simulink model "commandABT"  (R2023a)
settings: Solver=FixedStepAuto  StartTime=0.0  StopTime=inf  RelTol=1e-3  EnableMultiTasking=on
undefined symbols (not defined in the file or in its folder): Aw, I, Kp, Kpd, PWMcmdMono1, PWMcmdMono2, PWMcmdMono3, PWMcmdMono4, speedMono1, speedMono2, speedMono3, speedMono4
libraries: arduinolib x8, arduinosensorlib x2, sharedtransform x2, mspfiltlib x1, matrix_library x1
settings Model: ExtModeTrigDuration=2  Creator=C23Clement.Azpiroz.F  LastModifiedBy=Clément
settings OptimizationCC: EnhancedBackFolding=on  PassReuseOutputArgsAs=Individual arguments  ZeroExternalMemoryAtStartup=off  ZeroInternalMemoryAtStartup=off  MaxStackSize=64  OptimizeBlockOrder=speed  DifferentSizesBufferReuse=on  OptimizationCustomize=off  EfficientTunableParamExpr=on
settings DebuggingCC: ParameterTunabilityLossMsg=error
settings HardwareCC: ProdBitPerPointer=32  ProdBitPerSizeT=32  ProdBitPerPtrDiffT=32  ProdLargestAtomicInteger=Long  ProdLargestAtomicFloat=Double  ProdWordSize=32  ProdHWDeviceType=ARM Compatible->ARM Cortex  UseEmbeddedCoderFeatures=off
settings SFSimCC: MATLABDynamicMemAlloc=off
settings RTWCC: Description=Embedded Coder  SystemTargetFile=ert.tlc  HardwareBoard=Arduino MKR1000  TemplateMakefile=ert_default_tmf  Toolchain=Arduino ARM  BuildConfiguration=Faster Runs
settings CodeAppCC: ForceParamTrailComments=on  OperatorAnnotations=on  SimulinkDataObjDesc=on  SFDataObjDesc=on  InsertBlockDesc=on
settings ERTTargetCC: SupportContinuousTime=on  SupportNonInlinedSFcns=on  SupportVariableSizeSignals=on  ExtModeTransport=2  ExtModeStaticAlloc=on  ExtModeAutomaticAllocSize=off  ExtModeStaticAllocSize=8192  ExtModeMexFile=ext_xcp  ExtModeIntrfLevel=Level2 - Open  ERTSrcFileBannerTemplate=codertarget_code_template.cgt  ERTHdrFileBannerTemplate=codertarget_code_template.cgt  ERTDataSrcFileTemplate=codertarget_code_template.cgt  ERTDataHdrFileTemplate=codertarget_code_template.cgt

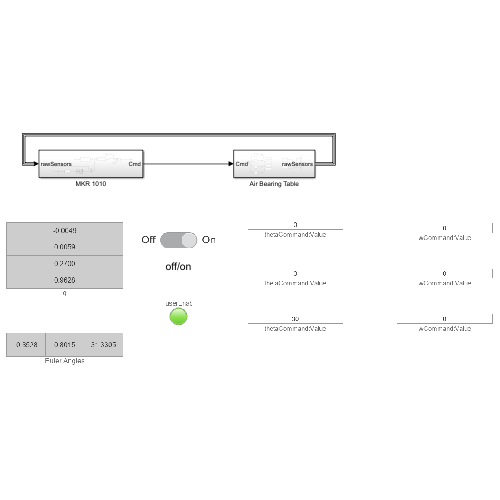
[thumbnail: Simulink's stored preview of the top-level diagram]
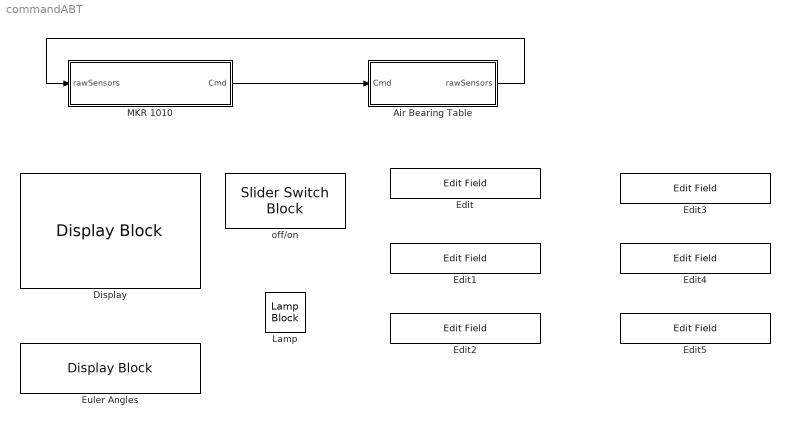
== system commandABT ==
  Air Bearing Table : Subsystem
  Display : DisplayBlock  LabelPosition=Bottom  Transparency=1
  Edit{,1..5} (6 alike) : EditField  LabelPosition=Bottom  ShowInitialText=on  Alignment=Center
  Euler Angles : DisplayBlock  LabelPosition=Bottom  Transparency=1
  Lamp : LampBlock
  MKR 1010 : Subsystem
  off/on : SliderSwitchBlock  LabelPosition=Hide
      settings: Values={{'Off', 'On'}, [0 1]}
  wires:
  Air Bearing Table/1(rawSensors) -> MKR 1010/1(rawSensors)
  MKR 1010/1(Cmd) -> Air Bearing Table/1(Cmd)

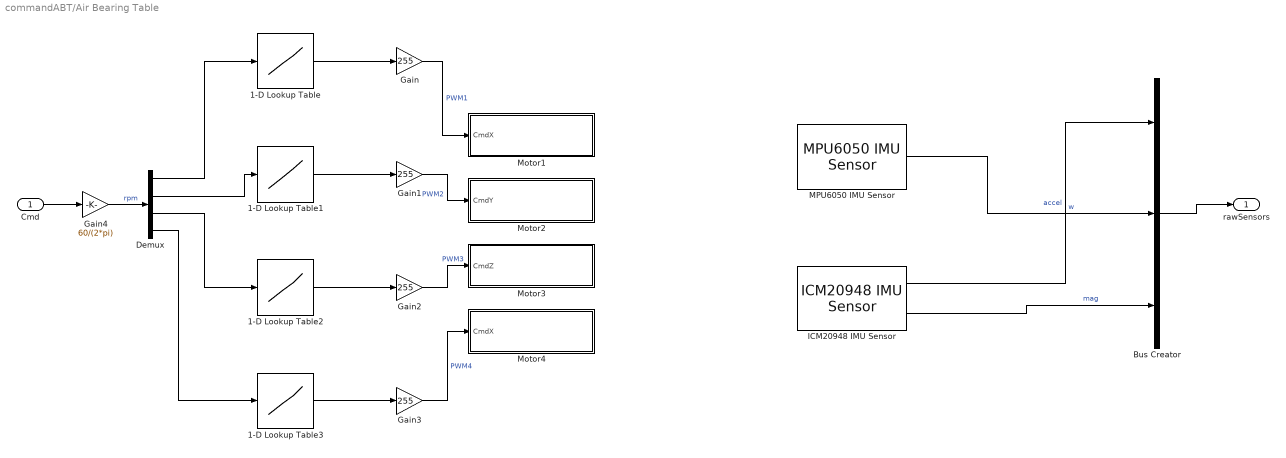
== system commandABT/Air Bearing Table ==
  Cmd : Inport
  1-D Lookup Table : Lookup_n-D  NumberOfTableDimensions=1  BreakpointsForDimension1=speedMono1  Table=PWMcmdMono1  InternalRulePriority=Speed  RndMeth=Simplest
  1-D Lookup Table1 : Lookup_n-D  NumberOfTableDimensions=1  BreakpointsForDimension1=speedMono2  Table=PWMcmdMono2  InternalRulePriority=Speed  RndMeth=Simplest
  1-D Lookup Table2 : Lookup_n-D  NumberOfTableDimensions=1  BreakpointsForDimension1=speedMono3  Table=PWMcmdMono3  InternalRulePriority=Speed  RndMeth=Simplest
  1-D Lookup Table3 : Lookup_n-D  NumberOfTableDimensions=1  BreakpointsForDimension1=speedMono4  Table=PWMcmdMono4  InternalRulePriority=Speed  RndMeth=Simplest
  Bus Creator : BusCreator  Inputs=3
  Demux : Demux
  Gain{,1..3} (4 alike) : Gain  Gain=255
  Gain4 : Gain  Gain=60/(2*pi)
  ICM20948 IMU Sensor : arduinosensorlib/ICM20948 IMU Sensor  I2CAddress=0x69  BitRate=1000000  EnableDRDY=off  InterruptType=Active high  IsActiveAccel=on  IsActiveGyro=off  IsActiveMag=on  IsActiveTemp=off  IsActiveStatus=off  IsActiveTimeStamp=off  AccelerometerRange=+/-2g  AccelerometerODR=1125  AccelerometerBW=23.9 Hz  GyroscopeRange=+/-250 dps  GyroscopeODR=1125  GyroscopeBW=23.9 Hz  MagnetometerODR=100 Hz  TemperatureBW=34.1 Hz  DataType=double  spf=1  SampleTime=0.1  QueueSizeFactor=1
  MPU6050 IMU Sensor : arduinosensorlib/MPU6050 IMU Sensor  SlaveAddress=0x68  Accel=off  AngularRate=on  Temperature=off  Status=off  Timestamp=off  EulerAngles=off  Quat=off  AccelRange=2G  GyroRange=250 dps  DmpOdr=200 Hz  Dlpf=Accelerometer: 184Hz, Gyroscope: 188Hz  spf=1  SampleTime=0.1  QueueSizeFactor=1
  Motor1 : Subsystem
  Motor2 : Subsystem
  Motor3 : Subsystem
  Motor4 : Subsystem
  rawSensors : Outport
  wires:
  Bus Creator/1 -> rawSensors/1
  Demux/1 -> 1-D Lookup Table/1
  Gain/1 -> Motor1/1(CmdX)  "PWM1"
  Cmd/1 -> Gain4/1
  1-D Lookup Table2/1 -> Gain2/1
  1-D Lookup Table1/1 -> Gain1/1
  Gain4/1 -> Demux/1  "rpm"
  Gain2/1 -> Motor3/1(CmdZ)  "PWM3"
  Gain3/1 -> Motor4/1(CmdX)  "PWM4"
  Demux/4 -> 1-D Lookup Table3/1
  Demux/3 -> 1-D Lookup Table2/1
  1-D Lookup Table/1 -> Gain/1
  Gain1/1 -> Motor2/1(CmdY)  "PWM2"
  Demux/2 -> 1-D Lookup Table1/1
  1-D Lookup Table3/1 -> Gain3/1
  MPU6050 IMU Sensor/1 -> Bus Creator/2  "w"
  ICM20948 IMU Sensor/1 -> Bus Creator/1  "accel"
  ICM20948 IMU Sensor/2 -> Bus Creator/3  "mag"

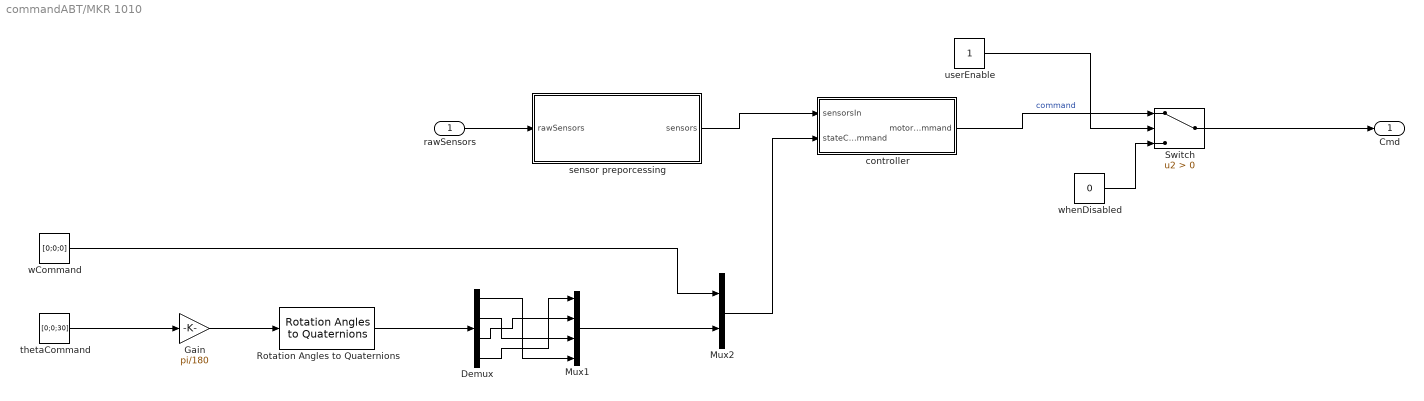
== system commandABT/MKR 1010 ==
  rawSensors : Inport
  Demux : Demux
  Gain : Gain  Gain=pi/180
  Mux1 : Mux
  Mux2 : Mux  Inputs=2
  Rotation Angles to Quaternions : sharedtransform/Rotation Angles to Quaternions  rotationOrder=ZYX  aMode=aMode
  Switch : Switch  Criteria=u2 > Threshold  SaturateOnIntegerOverflow=off  InputSameDT=off
  controller : Subsystem
  sensor preporcessing : Subsystem
  thetaCommand : Constant  Value=[0;0;30]
  userEnable : Constant
  wCommand : Constant  Value=[0;0;0]
  whenDisabled : Constant  Value=0
  Cmd : Outport
  wires:
  rawSensors/1 -> sensor preporcessing/1(rawSensors)
  userEnable/1 -> Switch/2
  sensor preporcessing/1(sensors) -> controller/1(sensorsIn)
  whenDisabled/1 -> Switch/3
  controller/1(motorCommand) -> Switch/1  "command"
  Switch/1 -> Cmd/1
  Demux/1 -> Mux1/4
  Demux/4 -> Mux1/1
  Demux/2 -> Mux1/3
  Demux/3 -> Mux1/2
  Gain/1 -> Rotation Angles to Quaternions/1
  Rotation Angles to Quaternions/1 -> Demux/1
  thetaCommand/1 -> Gain/1
  wCommand/1 -> Mux2/1
  Mux1/1 -> Mux2/2
  Mux2/1 -> controller/2(stateCommand)

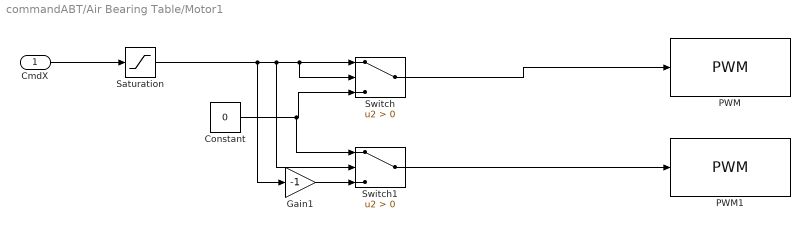
== system commandABT/Air Bearing Table/Motor1 ==
  CmdX : Inport
  Constant : Constant  Value=0
  Gain1 : Gain  Gain=-1
  PWM : arduinolib/PWM  pinNumber=2  frequencyType=Default  desiredFrequency=490.2  achievableFrequency=490.2
  PWM1 : arduinolib/PWM  pinNumber=3  frequencyType=Default  desiredFrequency=490.2  achievableFrequency=490.2
  Saturation : Saturate  UpperLimit=255  LowerLimit=-255
  Switch : Switch  Criteria=u2 > Threshold  SaturateOnIntegerOverflow=off  InputSameDT=off
  Switch1 : Switch  Criteria=u2 > Threshold  SaturateOnIntegerOverflow=off  InputSameDT=off
  wires:
  Switch1/1 -> PWM1/1
  CmdX/1 -> Saturation/1
  Switch/1 -> PWM/1
  Saturation/1 -> Gain1/1, Switch/1, Switch/2, Switch1/2
  Constant/1 -> Switch1/1, Switch/3
  Gain1/1 -> Switch1/3

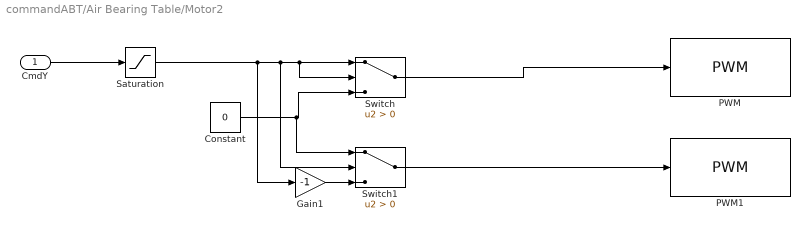
== system commandABT/Air Bearing Table/Motor2 ==
  CmdY : Inport
  Constant : Constant  Value=0
  Gain1 : Gain  Gain=-1
  PWM : arduinolib/PWM  pinNumber=4  frequencyType=Default  desiredFrequency=490.2  achievableFrequency=490.2
  PWM1 : arduinolib/PWM  pinNumber=5  frequencyType=Default  desiredFrequency=490.2  achievableFrequency=490.2
  Saturation : Saturate  UpperLimit=255  LowerLimit=-255
  Switch : Switch  Criteria=u2 > Threshold  SaturateOnIntegerOverflow=off  InputSameDT=off
  Switch1 : Switch  Criteria=u2 > Threshold  SaturateOnIntegerOverflow=off  InputSameDT=off
  wires:
  Switch1/1 -> PWM1/1
  CmdY/1 -> Saturation/1
  Switch/1 -> PWM/1
  Saturation/1 -> Gain1/1, Switch/1, Switch/2, Switch1/2
  Constant/1 -> Switch1/1, Switch/3
  Gain1/1 -> Switch1/3

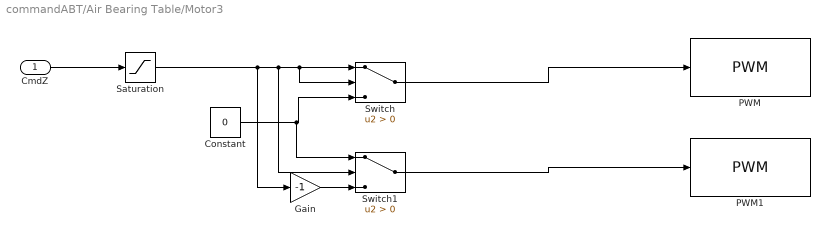
== system commandABT/Air Bearing Table/Motor3 ==
  CmdZ : Inport
  Constant : Constant  Value=0
  Gain : Gain  Gain=-1
  PWM : arduinolib/PWM  pinNumber=0  frequencyType=Default  desiredFrequency=490.2  achievableFrequency=490.2
  PWM1 : arduinolib/PWM  pinNumber=1  frequencyType=Default  desiredFrequency=490.2  achievableFrequency=490.2
  Saturation : Saturate  UpperLimit=255  LowerLimit=-255
  Switch : Switch  Criteria=u2 > Threshold  SaturateOnIntegerOverflow=off  InputSameDT=off
  Switch1 : Switch  Criteria=u2 > Threshold  SaturateOnIntegerOverflow=off  InputSameDT=off
  wires:
  Switch1/1 -> PWM1/1
  CmdZ/1 -> Saturation/1
  Switch/1 -> PWM/1
  Constant/1 -> Switch1/1, Switch/3
  Saturation/1 -> Gain/1, Switch1/2, Switch/2, Switch/1
  Gain/1 -> Switch1/3

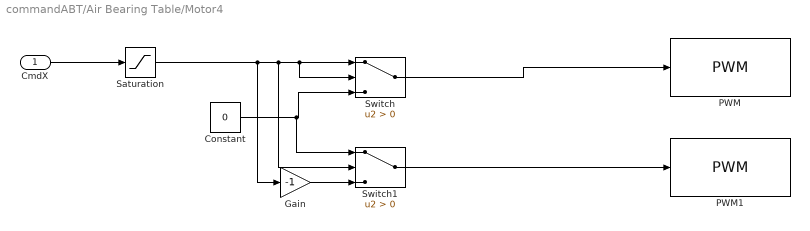
== system commandABT/Air Bearing Table/Motor4 ==
  CmdX : Inport
  Constant : Constant  Value=0
  Gain : Gain  Gain=-1
  PWM : arduinolib/PWM  pinNumber=6  frequencyType=Default  desiredFrequency=490.2  achievableFrequency=490.2
  PWM1 : arduinolib/PWM  pinNumber=7  frequencyType=Default  desiredFrequency=490.2  achievableFrequency=490.2
  Saturation : Saturate  UpperLimit=255  LowerLimit=-255
  Switch : Switch  Criteria=u2 > Threshold  SaturateOnIntegerOverflow=off  InputSameDT=off
  Switch1 : Switch  Criteria=u2 > Threshold  SaturateOnIntegerOverflow=off  InputSameDT=off
  wires:
  Switch1/1 -> PWM1/1
  CmdX/1 -> Saturation/1
  Switch/1 -> PWM/1
  Constant/1 -> Switch1/1, Switch/3
  Saturation/1 -> Gain/1, Switch1/2, Switch/2, Switch/1
  Gain/1 -> Switch1/3

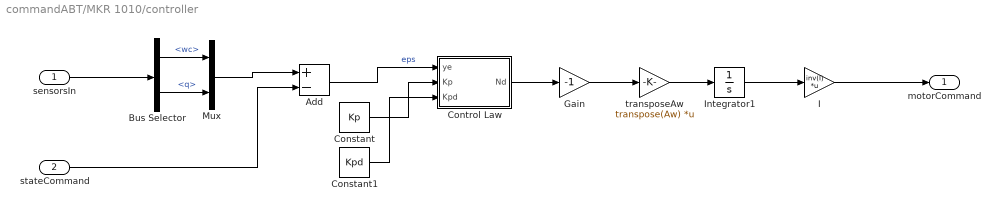
== system commandABT/MKR 1010/controller ==
  sensorsIn : Inport
  stateCommand : Inport  Port=2
  Add : Sum  Inputs=+-
  Bus Selector : BusSelector  OutputSignals=wc,q
  Constant : Constant  Value=Kp
  Constant1 : Constant  Value=Kpd
  Control Law : MATLAB Function  TreatAsAtomicUnit=on
  Gain : Gain  Gain=-1
  I : Gain  Gain=inv(I)  Multiplication=Matrix(K*u)
  Integrator1 : Integrator  InitialCondition=[0.01; 0.01; 0.01; 0.01]
  Mux : Mux  Inputs=2
  transposeAw : Gain  Gain=transpose(Aw)  Multiplication=Matrix(K*u)
  motorCommand : Outport
  wires:
  sensorsIn/1 -> Bus Selector/1
  Bus Selector/1 -> Mux/1  "<wc>"
  Bus Selector/2 -> Mux/2  "<q>"
  Mux/1 -> Add/1
  stateCommand/1 -> Add/2
  Add/1 -> Control Law/1(ye)  "eps"
  Constant/1 -> Control Law/2(Kp)
  Constant1/1 -> Control Law/3(Kpd)
  Control Law/1(Nd) -> Gain/1
  transposeAw/1 -> Integrator1/1
  Integrator1/1 -> I/1
  I/1 -> motorCommand/1
  Gain/1 -> transposeAw/1

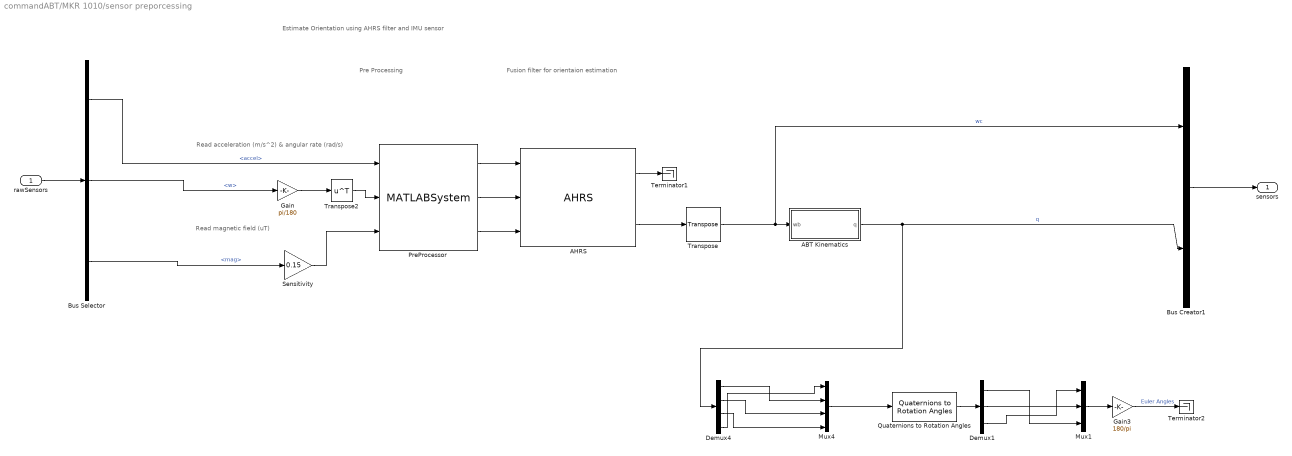
== system commandABT/MKR 1010/sensor preporcessing ==
  note: Fusion filter for orientaion estimation
  note: Read  acceleration (m/s^2) &
      | angular rate (rad/s)
  note: Read magnetic field (uT)
  note: Estimate Orientation using AHRS filter and IMU sensor
  note: Pre Processing
  rawSensors : Inport
  ABT Kinematics : Subsystem
  AHRS : mspfiltlib/AHRS  DispRefFrame=ENU  DecimationFactor=1  InitialProcessNoise=ahrsfilter.defaultProcessNoise  OrientationFormat=quaternion  SimulateUsing=Interpreted execution  AccelerometerNoise=0.000134  GyroscopeNoise=1.38347e-6  MagnetometerNoise=0.45  GyroscopeDriftNoise=0.1e-30  LinearAccelerationNoise=0.0096236100000000012  MagneticDisturbanceNoise=0.5  LinearAccelerationDecayFactor=0.5  MagneticDisturbanceDecayFactor=0.5  ExpectedMagneticFieldStrength=50
  Bus Creator1 : BusCreator  Inputs=2
  Bus Selector : BusSelector  OutputSignals=accel,w,mag
  Demux1 : Demux  Outputs=3
  Demux4 : Demux
  Gain : Gain  Gain=pi/180
  Gain3 : Gain  Gain=180/pi
  Mux1 : Mux  Inputs=3
  Mux4 : Mux
  PreProcessor : MATLABSystem  System=PreProcessor  MagOffsets=[-3.7477,2.6230,9.3852]  AccelXAxisIndex=2  AccelXAxisSign=-  AccelYAxisIndex=1  AccelYAxisSign=-  AccelZAxisIndex=3  AccelZAxisSign=-  GyroXAxisIndex=2  GyroXAxisSign=+  GyroYAxisIndex=1  GyroYAxisSign=-  GyroZAxisIndex=3  GyroZAxisSign=+  MagXAxisIndex=2  MagXAxisSign=-  MagYAxisIndex=1  MagYAxisSign=-  MagZAxisIndex=3  MagZAxisSign=-
      mask Type: PreProcessor
      mask Display:
      | disp('PreProcessor');
      | port_label('input',1,'accel');
      | port_label('input',2,'gyro');
      | port_label('input',3,'mag');
      | port_label('output',1,'accel');
      | port_label('output',2,'gyro');
      | port_label('output',3,'mag');
  Quaternions to Rotation Angles : sharedtransform/Quaternions to Rotation Angles  rotationOrder=ZYX  aMode=aMode
  Sensitivity : Gain  Gain=0.15  OutDataTypeStr=double  LockScale=on
  Terminator1 : Terminator
  Terminator2 : Terminator
  Transpose : matrix_library/Transpose
  Transpose2 : Math  Operator=transpose
  sensors : Outport
  wires:
  rawSensors/1 -> Bus Selector/1
  Bus Creator1/1 -> sensors/1
  Demux1/1 -> Mux1/3
  Demux1/3 -> Mux1/1
  Mux1/1 -> Gain3/1
  Quaternions to Rotation Angles/1 -> Demux1/1
  ABT Kinematics/1(q) -> Bus Creator1/2, Demux4/1  "q"
  Demux1/2 -> Mux1/2
  Gain3/1 -> Terminator2/1  "Euler Angles"
  Demux4/1 -> Mux4/2
  Demux4/3 -> Mux4/4
  Demux4/4 -> Mux4/1
  Demux4/2 -> Mux4/3
  Mux4/1 -> Quaternions to Rotation Angles/1
  PreProcessor/1 -> AHRS/1
  Sensitivity/1 -> PreProcessor/3
  Bus Selector/2 -> Gain/1  "<w>"
  Transpose2/1 -> PreProcessor/2
  PreProcessor/3 -> AHRS/3
  Bus Selector/3 -> Sensitivity/1  "<mag>"
  AHRS/2 -> Transpose/1
  Gain/1 -> Transpose2/1
  PreProcessor/2 -> AHRS/2
  AHRS/1 -> Terminator1/1
  Bus Selector/1 -> PreProcessor/1  "<accel>"
  Transpose/1 -> Bus Creator1/1, ABT Kinematics/1(wb)  "wc"

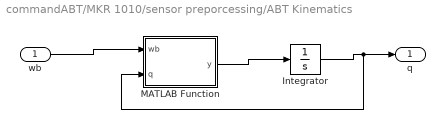
== system commandABT/MKR 1010/sensor preporcessing/ABT Kinematics ==
  wb : Inport
  Integrator : Integrator  InitialCondition=[0; 0; 0; 1]
  MATLAB Function : MATLAB Function  TreatAsAtomicUnit=on
  q : Outport
  wires:
  wb/1 -> MATLAB Function/1(wb)
  MATLAB Function/1(y) -> Integrator/1
  Integrator/1 -> MATLAB Function/2(q), q/1

== matlab function commandABT/MKR 1010/sensor preporcessing/ABT Kinematics/MATLAB Function ==
  data: wb input; y output; q input
function y = fcn(wb,q)
W = [0, wb(3), -wb(2), wb(1); -wb(3), 0, wb(1), wb(2); wb(2), -wb(1), 0, wb(3); -wb(1), -wb(2), -wb(3), 0]
y = 0.5*W*q

== matlab function commandABT/MKR 1010/controller/Control Law ==
  data: ye input; Nd output; Kp input; Kpd input
function Nd = fcn(ye, Kp, Kpd)

Nd = -[Kpd Kp]*ye(1:6);
